simulink model "check_ndtm_latinclination"  (R2018b)
settings: configuration reference "Physics" (kept outside this file)
libraries: simulink x1
settings Model: DataDictionary=check_ndtm.sldd  OrderedModelArguments=off  Creator=wischnewski  LastModifiedBy=ga25xiw

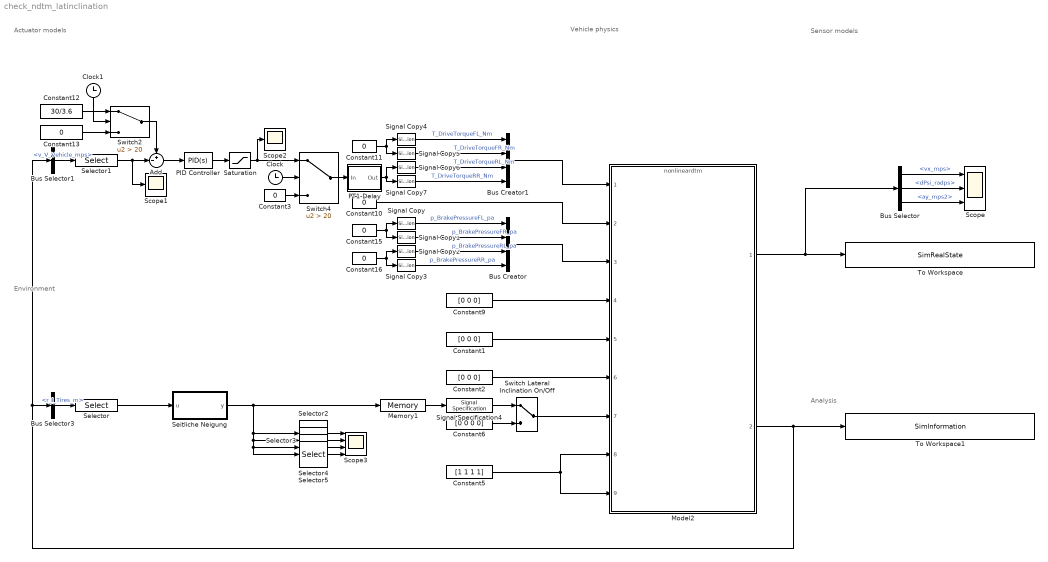
== system check_ndtm_latinclination ==
  note: Actuator models
  note: Vehicle physics
  note: Environment
  note: Analysis
  note: Sensor models
  Add : Sum  Inputs=+-|
  Bus Creator : BusCreator  Inputs=4  OutDataTypeStr=Bus: BrakePressure_Pa
  Bus Creator1 : BusCreator  Inputs=4  OutDataTypeStr=Bus: DriveTorque_Nm
  Bus Selector : BusSelector  OutputSignals=vx_mps,dPsi_radps,ay_mps2
  Bus Selector1 : BusSelector  OutputSignals=Vehicle.v_V_Vehicle_mps
  Bus Selector3 : BusSelector  OutputSignals=Wheel.r_I_Tires_m
  Clock : Clock
  Clock1 : Clock
  Constant1 : Constant  Value=[0 0 0]
  Constant{3,10..11,13,15..16} (6 alike) : Constant  Value=0
  Constant12 : Constant  Value=30/3.6
  Constant2 : Constant  Value=[0 0 0]
  Constant5 : Constant  Value=[1 1 1 1]
  Constant6 : Constant  Value=[0 0 0 0]
  Constant9 : Constant  Value=[0 0 0]
  Memory1 : Memory
  Model2 : ModelReference  ModelNameDialog=nonlineardtm  ParameterArgumentNames=x0_vehiclepose  ParameterArgumentValues=[0,0,0]  UsingDefaultArgumentValue=0  SimulationMode=Normal  ModelReferenceVersion=1.633
  PID Controller : simulink/Continuous/PID Controller  Controller=PID  Form=Parallel  TimeDomain=Continuous-time  SampleTime=-1  IntegratorMethod=Forward Euler  FilterMethod=Forward Euler  ControllerParametersSource=internal  P=750  I=1  D=0  UseFilter=on  N=100  TunerSelectOption=Transfer Function Based (PID Tuner App)  InitialConditionSource=internal  InitialConditionForIntegrator=0  InitialConditionForFilter=0  DifferentiatorICPrevScaledInput=0  ExternalReset=none  TrackingMode=off  Kt=1  LimitOutput=off  UpperSaturationLimit=inf  LowerSaturationLimit=-inf  LinearizeAsGain=on  AntiWindupMode=none  Kb=1  POutMin=[]  POutMax=[]  IOutMin=[]  IOutMax=[]  DOutMin=[]  DOutMax=[]  NOutMin=[]  NOutMax=[]  SumOutMin=[]  SumOutMax=[]  SaturationOutMin=[]  SaturationOutMax=[]  PParamMin=[]  PParamMax=[]  IParamMin=[]  IParamMax=[]  DParamMin=[]  DParamMax=[]  NParamMin=[]  NParamMax=[]  KbParamMin=[]  KbParamMax=[]  KtParamMin=[]  KtParamMax=[]  KbOutMin=[]  KbOutMax=[]  KtOutMin=[]  KtOutMax=[]  IntegratorOutMin=[]  IntegratorOutMax=[]  FilterOutMin=[]  FilterOutMax=[]  SumI1OutMin=[]  SumI1OutMax=[]  SumI2OutMin=[]  SumI2OutMax=[]  SumI3OutMin=[]  SumI3OutMax=[]  SumI4OutMin=[]  SumI4OutMax=[]  SumDOutMin=[]  SumDOutMax=[]  DifferentiatorOutMin=[]  DifferentiatorOutMax=[]  FilterDiffOutCoefMin=[]  FilterDiffOutCoefMax=[]  ReciprocalOutMin=[]  ReciprocalOutMax=[]  SumDenOutMin=[]  SumDenOutMax=[]  SumNumOutMin=[]  SumNumOutMax=[]  DivideOutMin=[]  DivideOutMax=[]  IntegratorContinuousStateAttributes=''  IntegratorStateMustResolveToSignalObject=off  IntegratorRTWStateStorageClass=Auto  FilterContinuousStateAttributes=''  FilterStateMustResolveToSignalObject=off  FilterRTWStateStorageClass=Auto  ParallelPVariant=InternalParameters  IdealPVariant=Disabled  IVariant=InternalParameters  DVariant=InternalParameters  IntegratorVariant=Continuous  SatVariant=Disabled  AWVariant=Passthrough  PCopyVariant=Disabled  TRVariant=Disabled  FdbkBlocksVariant=Forward  IdealPFdbkVariant=Disabled  SatFdbkVariant=Disabled  DerivativeFilterVariant=ContFilter  NVariant=InternalParameters  NCopyVariant=Disabled  FilterICVariant=InternalICsFilter  IntegratorICVariant=InternalICs  ExternalResetVariant=Disabled  TRSumVariant=Passthrough  SumFdbkVariant=Disabled  SumVariant=Sum_PID
  PT1-Delay : Subsystem
  Saturation : Saturate  UpperLimit=500  LowerLimit=0
  Scope : Scope  NumInputPorts=3
  Scope1 : Scope
  Scope2 : Scope
  Scope3 : Scope  NumInputPorts=4
  Seitliche Neigung : MATLAB Function  TreatAsAtomicUnit=on
  Selector : Selector  NumberOfDimensions=2  InputPortWidth=3  IndexOptions=Index vector (dialog),Select all  Indices=1,1  OutputSizes=1,1
  Selector1 : Selector  InputPortWidth=3  IndexOptions=Index vector (dialog)  Indices=1  OutputSizes=1
  Selector2 : Selector  InputPortWidth=4  IndexOptions=Index vector (dialog)  Indices=1  OutputSizes=1
  Selector3 : Selector  InputPortWidth=4  IndexOptions=Index vector (dialog)  Indices=2  OutputSizes=1
  Selector4 : Selector  InputPortWidth=4  IndexOptions=Index vector (dialog)  Indices=3  OutputSizes=1
  Selector5 : Selector  InputPortWidth=4  IndexOptions=Index vector (dialog)  Indices=4  OutputSizes=1
  Signal Copy{,1..7} (8 alike) : SignalConversion  OverrideOpt=off
  Signal Specification4 : SignalSpecification  Dimensions=[1 4]
  Switch Lateral Inclination On/Off : ManualSwitch
  Switch2 : Switch  Criteria=u2 > Threshold  Threshold=20
  Switch4 : Switch  Criteria=u2 > Threshold  Threshold=20
  To Workspace : ToWorkspace  VariableName=SimRealState  SaveFormat=Timeseries  SampleTime=-1
  To Workspace1 : ToWorkspace  VariableName=SimInformation  SaveFormat=Timeseries  SampleTime=-1
  wires:
  Bus Selector/1 -> Scope/1  "<vx_mps>"
  Bus Selector/2 -> Scope/2  "<dPsi_radps>"
  Bus Selector/3 -> Scope/3  "<ay_mps2>"
  Model2/1 -> Bus Selector/1, To Workspace/1
  Constant9/1 -> Model2/4
  Constant1/1 -> Model2/5
  Constant2/1 -> Model2/6
  Constant5/1 -> Model2/8, Model2/9
  Bus Selector3/1 -> Selector/1  "<r_I_Tires_m>"
  Constant6/1 -> Switch Lateral Inclination On/Off/2
  Model2/2 -> To Workspace1/1, Bus Selector1/1, Bus Selector3/1
  Switch Lateral Inclination On/Off/1 -> Model2/7
  Seitliche Neigung/1(y) -> Memory1/1, Selector2/1, Selector3/1, Selector5/1, Selector4/1
  Bus Selector1/1 -> Selector1/1  "<v_V_Vehicle_mps>"
  Selector1/1 -> Scope1/1, Add/2
  PID Controller/1 -> Saturation/1
  Add/1 -> PID Controller/1
  Constant12/1 -> Switch2/1
  Saturation/1 -> Switch4/1, Scope2/1
  Clock/1 -> Switch4/2
  Constant3/1 -> Switch4/3
  Constant13/1 -> Switch2/3
  Clock1/1 -> Switch2/2
  Switch2/1 -> Add/1
  Signal Specification4/1 -> Switch Lateral Inclination On/Off/1
  Switch4/1 -> PT1-Delay/1(In)
  Memory1/1 -> Signal Specification4/1
  Selector2/1 -> Scope3/1
  Selector3/1 -> Scope3/2
  Selector4/1 -> Scope3/3
  Selector5/1 -> Scope3/4
  Selector/1 -> Seitliche Neigung/1(u)
  Signal Copy2/1 -> Bus Creator/3  "p_BrakePressureRL_pa"
  PT1-Delay/1(Out) -> Signal Copy6/1, Signal Copy7/1
  Signal Copy/1 -> Bus Creator/1  "p_BrakePressureFL_pa"
  Signal Copy1/1 -> Bus Creator/2  "p_BrakePressureFR_pa"
  Bus Creator/1 -> Model2/3
  Constant10/1 -> Model2/2
  Bus Creator1/1 -> Model2/1
  Signal Copy5/1 -> Bus Creator1/2  "T_DriveTorqueFR_Nm"
  Signal Copy7/1 -> Bus Creator1/4  "T_DriveTorqueRR_Nm"
  Signal Copy4/1 -> Bus Creator1/1  "T_DriveTorqueFL_Nm"
  Signal Copy6/1 -> Bus Creator1/3  "T_DriveTorqueRL_Nm"
  Constant16/1 -> Signal Copy3/1, Signal Copy2/1
  Signal Copy3/1 -> Bus Creator/4  "p_BrakePressureRR_pa"
  Constant11/1 -> Signal Copy4/1, Signal Copy5/1
  Constant15/1 -> Signal Copy1/1, Signal Copy/1

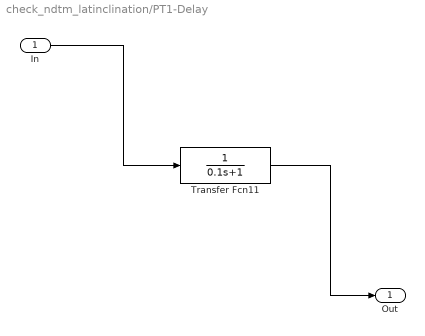
== system check_ndtm_latinclination/PT1-Delay ==
  In : Inport
  Transfer Fcn11 : TransferFcn  Denominator=[0.1 1]
  Out : Outport
  wires:
  In/1 -> Transfer Fcn11/1
  Transfer Fcn11/1 -> Out/1

== matlab function check_ndtm_latinclination/Seitliche Neigung ==
  data: u input; y output
function y = fcn(u)

profil=zeros(1,4);

for i=1:4
    
if u(i)>100 && u(i)<500
    profil(i)=-0.05-0.05*sin(pi/400*(u(i)-300));
elseif u(i)>=500 && u(i)<=700
    profil(i)=-0.1;
elseif u(i)>700 && u(i)<1100
    profil(i)=-0.05+0.05*sin(pi/400*(u(i)-900));
else
    profil(i)=0;
end    

profil(1)=0;
profil(3)=0;
y=profil;

end
